simulink model "chap6_4"  (Simulink 5.0)
settings: Solver=ode5  StartTime=0.0  StopTime=500  FixedStep=1  RelTol=1e-3

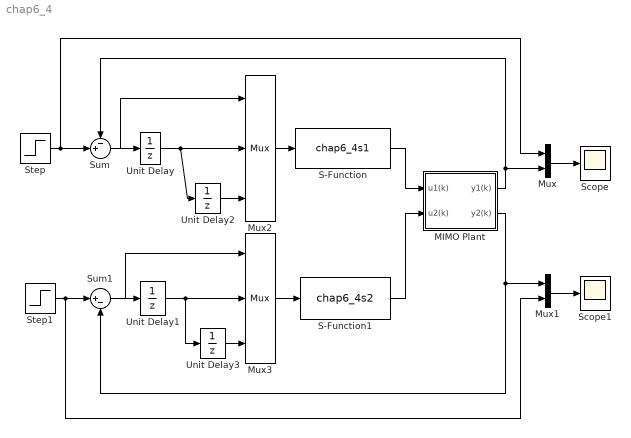
== system chap6_4 ==
  MIMO Plant : Subsystem
  Mux : Mux  Inputs=2
  Mux1 : Mux  Inputs=2
  Mux2 : Mux  Inputs=3
  Mux3 : Mux  Inputs=3
  S-Function : S-Function  FunctionName=chap6_4s1
  S-Function1 : S-Function  FunctionName=chap6_4s2
  Scope : Scope
      settings: TimeRange=1500  YMin=0  YMax=1  SaveName=yy  DataFormat=Array
  Scope1 : Scope
      settings: TimeRange=1500  YMin=0  YMax=1  SaveName=yy1  DataFormat=Array
  Step : Step  SampleTime=1
  Step1 : Step  SampleTime=1
  Sum : Sum  Inputs=-+|  SaturateOnIntegerOverflow=on
  Sum1 : Sum  Inputs=|+-  SaturateOnIntegerOverflow=on
  Unit Delay{,1..3} (4 alike) : UnitDelay
  wires:
  MIMO Plant/2(y2(k)) -> Sum1/2, Mux1/1
  MIMO Plant/1(y1(k)) -> Sum/1, Mux/2
  S-Function/1 -> MIMO Plant/1(u1(k))
  S-Function1/1 -> MIMO Plant/2(u2(k))
  Step1/1 -> Sum1/1, Mux1/2
  Step/1 -> Sum/2, Mux/1
  Sum/1 -> Mux2/1, Unit Delay/1
  Sum1/1 -> Mux3/1, Unit Delay1/1
  Mux/1 -> Scope/1
  Mux1/1 -> Scope1/1
  Mux2/1 -> S-Function/1
  Unit Delay/1 -> Mux2/2, Unit Delay2/1
  Mux3/1 -> S-Function1/1
  Unit Delay1/1 -> Mux3/2, Unit Delay3/1
  Unit Delay2/1 -> Mux2/3
  Unit Delay3/1 -> Mux3/3

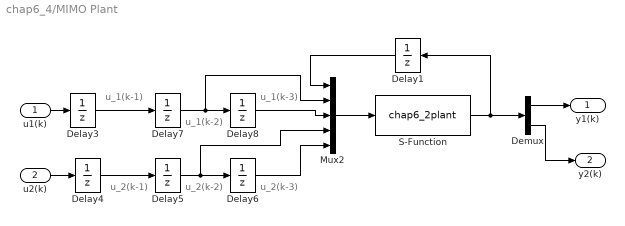
== system chap6_4/MIMO Plant ==
  note: u_1(k-1)
  note: u_1(k-2)
  note: u_1(k-3)
  note: u_2(k-1)
  note: u_2(k-2)
  note: u_2(k-3)
  u1(k) : Inport
  u2(k) : Inport  Port=2
  Delay1 : UnitDelay  Orientation=left  SampleTime=-1
  Delay{3..8} (6 alike) : UnitDelay  SampleTime=-1
  Demux : Demux  Outputs=2
  Mux2 : Mux  Inputs=5
  S-Function : S-Function  FunctionName=chap6_2plant  Parameters=1
  y1(k) : Outport
  y2(k) : Outport  Port=2
  wires:
  Delay3/1 -> Delay7/1
  Delay7/1 -> Delay8/1, Mux2/2
  u1(k)/1 -> Delay3/1
  Delay4/1 -> Delay5/1
  Delay5/1 -> Delay6/1, Mux2/4
  u2(k)/1 -> Delay4/1
  Delay6/1 -> Mux2/5
  Delay8/1 -> Mux2/3
  Mux2/1 -> S-Function/1
  Delay1/1 -> Mux2/1
  S-Function/1 -> Demux/1, Delay1/1
  Demux/1 -> y1(k)/1
  Demux/2 -> y2(k)/1
